simulink library "thc"  (R2021b)
settings: Solver=VariableStepAuto  StartTime=0.0  StopTime=10.0  RelTol=1e-3
undefined symbols (not defined in the file or in its folder): ATHC_APTCQA_X_C, ATHC_APTCQB_X_C, ATHC_dAy_X_C, ATHC_Qeq_X_kmh, ATHC_VbaseC_X_C, ATHC_VbaseC_Y_W, ATHC_VbaseD_X_C, ATHC_VbaseH_X_C, KTHC_ACMaxMinT_sec, KTHC_aDeice_K, KTHC_AGSDefLv_K, KTHC_AGSLv1_K, KTHC_AGSLv2_K, KTHC_AGSLv3_K, KTHC_AGSLv4_K, KTHC_AGSLv5_K, KTHC_AirIntUpdateT_sec, KTHC_APTCOneZoneMax_W, KTHC_APTCPeriod_cnt, KTHC_APTCPWMEN_flg, KTHC_APTCQMaxC_W, KTHC_APTCQminC_W, KTHC_APTCQminD_W, KTHC_APTCQminRe1_W, KTHC_APTCQminRe_W, KTHC_APTCQoffT_cnt, KTHC_APTCQonT_cnt, KTHC_APTCRiLeMaxDff_W, KTHC_APTCRiLeMinDff_W, KTHC_AutoWDTamb1_C, KTHC_AutoWDTamb2_C, KTHC_AutoWDTamb3_C, KTHC_BatCoolT_cnt, KTHC_BatInTempDef_C, KTHC_bDeice_K, KTHC_CompMaxDeice_rpm, KTHC_CompMinDeice_rpm, KTHC_CompSotxvOp_K, KTHC_CompSotxvOpLow_rpm, KTHC_CompSpdEXVUp1_rpm, KTHC_CompSpdEXVUp2_rpm, KTHC_CompSpdEXVUp3_rpm, KTHC_CompSpdEXVUp4_rpm, KTHC_CompSpdmax_rpm, KTHC_CompSpdmaxBC1_rpm, KTHC_CompSpdmaxBC_rpm, KTHC_CompSpdmid1_rpm, KTHC_CompSpdmid2_rpm, KTHC_CompSpdmid3_rpm, KTHC_CompSpdmid4_rpm, KTHC_CompSpdmid5_rpm, KTHC_CompSpdmid_rpm, KTHC_CompSpdmin_rpm, KTHC_DAPTCQ1_W, KTHC_DAPTCQ2_W, KTHC_DAPTCQ3_W, KTHC_DcChSetTemp_C, KTHC_DehumidityEN_flg, KTHC_DeiceCycTime_K, KTHC_DriveLevelWPTCBAH1_W ... (+403)
libraries: simulink x489
(part 13 of 18)

== system thc/THC/ThermalControl/THCM_Conctrl/EXV1Ctrl ==
  EXV1SHSetpoint : Inport
  PT_ Low_P1 : Inport  Port=2
  PT_ Low_T1 : Inport  Port=3
  BatteryMode : Inport  Port=4
  EXVOpen : Inport  Port=5
  ErrEXV1FroceOFF : Inport  Port=6
  HVBMTempMax : Inport  Port=7
  ChrgPlugSta : Inport  Port=8
  CompSpd : Inport  Port=9
  Chart : Stateflow chart  TreatAsAtomicUnit=on
  Compare To Constant : simulink/Logic and Bit Operations/Compare To Constant  relop===  const=1  OutDataTypeStr=boolean
  Compare To Constant1 : simulink/Logic and Bit Operations/Compare To Constant  relop===  const=1  OutDataTypeStr=boolean
  Compare To Constant2 : simulink/Logic and Bit Operations/Compare To Constant  relop===  const=6  OutDataTypeStr=boolean
  Compare To Constant3 : simulink/Logic and Bit Operations/Compare To Constant  relop===  const=6  OutDataTypeStr=boolean
  Compare To Constant4 : simulink/Logic and Bit Operations/Compare To Constant  relop===  const=2  OutDataTypeStr=boolean
  Constant : Constant  Value=0.1
  Constant1 : Constant  Value=538
  Constant{3,8..17} (11 alike) : Constant  Value=0
  Constant18 : Constant  Value=KTHC_EXVBlancePulse_K
  Constant19 : Constant  Value=ZERO_INT
  Constant2 : Constant  Value=38
  Constant20 : Constant  Value=KTHC_RefrigerantType_enum
  Constant21 : Constant  Value=KTHC_EXV1UplimLv1_K
  Constant22 : Constant  Value=KTHC_EXV1UplimLv2_K
  Constant23 : Constant  Value=KTHC_EXV1UplimLv3_K
  Constant24 : Constant  Value=KTHC_T3MinBC_C
  Constant25 : Constant  Value=KTHC_T4MinBC_C
  Constant26 : Constant  Value=KTHC_T2MaxBC_C
  Constant27 : Constant  Value=KTHC_T3MaxBC_C
  Constant28 : Constant  Value=KTHC_CompSpdEXVUp1_rpm
  Constant29 : Constant  Value=KTHC_CompSpdEXVUp2_rpm
  Constant30 : Constant  Value=KTHC_CompSpdEXVUp3_rpm
  Constant31 : Constant  Value=KTHC_CompSpdEXVUp4_rpm
  Constant4 : Constant  Value=KTHC_KpEXV1SH_K
  Constant5 : Constant  Value=KTHC_KiEXV1SHDeice_K
  Constant6 : Constant  Value=KTHC_KpEXV1SHDeice_K
  Constant7 : Constant  Value=KTHC_KiEXV1SH_K
  EXV1PIControl : Subsystem
  Equal : RelationalOperator  Operator=~=  OutDataTypeStr=boolean  RndMeth=Simplest
  Gain : Gain  Gain=1/1000
  Logical Operator : Logic  Operator=OR  AllPortsSameDT=off  OutDataTypeStr=boolean
  Logical Operator1 : Logic  AllPortsSameDT=off  OutDataTypeStr=boolean
  Logical Operator2 : Logic  Operator=OR  AllPortsSameDT=off  OutDataTypeStr=boolean
  Multiport Switch : MultiPortSwitch  Inputs=7  DiagnosticForDefault=None
  Multiport Switch1 : MultiPortSwitch  Inputs=7  DiagnosticForDefault=None
  Multiport Switch2 : MultiPortSwitch  DataPortOrder=Zero-based contiguous  zeroidx=on
  Product : Product
  R1234yf : Lookup_n-D  NumberOfTableDimensions=1  BreakpointsForDimension1=[0.03742 0.06237 0.09906 0.11778 0.15092 0.1909 0.2386 0.29495 0.36092 0.43753 0.52583 0.6269 0.74189 0.87197 1.0184 1.3023]  Table=[-50 -40 -30 -26 -20 -14 -8 -2 4 10 16 22 28 34 40 50]  InternalRulePriority=Speed  RndMeth=Simplest  InputSameDT=on
  R134a : Lookup_n-D  NumberOfTableDimensions=1  BreakpointsForDimension1=[0.02945 0.05121 0.08438 0.10167 0.13273 0.17082 0.21693 0.27217 0.33766 0.41461 0.50425 0.60789 0.72688 0.86263 1.0166 1.31790]  Table=[-50 -40 -30 -26 -20 -14 -8 -2 4 10 16 22 28 34 40 50]  InternalRulePriority=Speed  RndMeth=Simplest  InputSameDT=on
  Relational Operator : RelationalOperator  Operator=<  OutDataTypeStr=boolean  RndMeth=Simplest
  Saturation : Saturate  UpperLimit=1  LowerLimit=0
  Sum : Sum  Inputs=|-+
  Sum1 : Sum  Inputs=|+-
  Sum2 : Sum  Inputs=|+-
  Sum3 : Sum  Inputs=|++
  Switch{,1..3} (4 alike) : Switch  Criteria=u2 > Threshold
  Unit Delay : UnitDelay  SampleTime=-1  HasFrameUpgradeWarning=on
  Unit Delay1 : UnitDelay  SampleTime=-1  HasFrameUpgradeWarning=on
  EXV1 : Outport
  VTHC_EXV1P_K : Outport  Port=2
  VTHC_EXV1I_K : Outport  Port=3
  VTHC_EXV1U_K : Outport  Port=4
  VTHC_EXV1e_K : Outport  Port=5
  wires:
  Constant20/1 -> Compare To Constant4/1
  R134a/1 -> Switch2/3
  Gain/1 -> R134a/1, R1234yf/1
  Compare To Constant4/1 -> Switch2/2
  R1234yf/1 -> Switch2/1
  BatteryMode/1 -> Switch1/3
  Switch1/1 -> [BatteryMode]
  ErrEXV1FroceOFF/1 -> Switch1/2
  Constant19/1 -> Switch1/1
  Unit Delay1/1 -> Multiport Switch2/3
  EXVOpen/1 -> Multiport Switch2/1
  Constant18/1 -> Multiport Switch2/4
  Switch3/1 -> Multiport Switch2/2
  [VTHC_KiEXV1SH_K] -> EXV1PIControl/4(VTHC_KiEXV1SH_K)
  Multiport Switch1/1 -> [VTHC_KiEXV1SH_K]
  [VTHC_KpEXV1SH_K] -> EXV1PIControl/3(VTHC_KpEXV1SH_K)
  Multiport Switch/1 -> [VTHC_KpEXV1SH_K]
  Constant17/1 -> Multiport Switch1/8
  Constant16/1 -> Multiport Switch1/6
  Constant15/1 -> Multiport Switch1/5
  Constant14/1 -> Multiport Switch1/4
  Constant13/1 -> Multiport Switch1/3
  Constant12/1 -> Multiport Switch/8
  Constant11/1 -> Multiport Switch/6
  Constant10/1 -> Multiport Switch/5
  Constant9/1 -> Multiport Switch/4
  Constant8/1 -> Multiport Switch/3
  [BatteryMode] -> Multiport Switch1/1
  Constant7/1 -> Multiport Switch1/2
  Constant5/1 -> Multiport Switch1/7
  Constant6/1 -> Multiport Switch/7
  Constant4/1 -> Multiport Switch/2
  [BatteryMode] -> Multiport Switch/1
  Logical Operator2/1 -> Switch/2
  Compare To Constant3/1 -> Logical Operator2/2
  Compare To Constant1/1 -> Logical Operator2/1
  Logical Operator1/1 -> EXV1PIControl/2(Reset)
  Logical Operator/1 -> Logical Operator1/2
  Equal/1 -> Logical Operator1/1
  Compare To Constant2/1 -> Logical Operator/2
  Compare To Constant/1 -> Logical Operator/1
  Unit Delay/1 -> Equal/1
  [BatteryMode] -> Equal/2, Compare To Constant2/1, Compare To Constant/1, Unit Delay/1
  EXV1PIControl/2(VTHC_EXV1I_K) -> VTHC_EXV1I_K/1
  EXV1PIControl/1(VTHC_EXV1P_K) -> VTHC_EXV1P_K/1
  PT_ Low_T1/1 -> Sum/2  "Tlow1"
  Sum2/1 -> Saturation/1  "0.1-U"
  Constant2/1 -> Sum3/1
  Constant/1 -> Sum2/1
  Product/1 -> Sum3/2
  Saturation/1 -> Product/1  "EXV1%"
  Switch2/1 -> Sum/1  "Tsat_low1"
  EXV1SHSetpoint/1 -> Sum1/1  "SetSH"
  Multiport Switch2/1 -> EXV1/1, Unit Delay1/1  "EXV1_Pulse"
  EXV1PIControl/3(VTHC_EXV1U_K) -> Sum2/2, VTHC_EXV1U_K/1  "U"
  Sum/1 -> Sum1/2  "SH"
  PT_ Low_P1/1 -> Gain/1  "Plow1(kpa)"
  Constant3/1 -> Switch/3
  [BatteryMode] -> Compare To Constant1/1, Compare To Constant3/1
  Constant1/1 -> Product/2
  Sum1/1 -> EXV1PIControl/1(x), VTHC_EXV1e_K/1  "e"
  Sum3/1 -> Switch/1
  Relational Operator/1 -> Switch3/2
  Switch/1 -> Switch3/1, Relational Operator/1
  [VTHC_EXV1UplimPulse_K] -> Switch3/3, Relational Operator/2
  HVBMTempMax/1 -> Chart/2(HVBMTempMax)
  ChrgPlugSta/1 -> Chart/3(ChrgPlugSta)
  CompSpd/1 -> Chart/4(CompSpd)
  Constant21/1 -> Chart/5(KTHC_EXV1UplimLv1_K)
  Constant22/1 -> Chart/6(KTHC_EXV1UplimLv2_K)
  Constant23/1 -> Chart/7(KTHC_EXV1UplimLv3_K)
  Constant24/1 -> Chart/8(KTHC_T3MinBC_C)
  Constant25/1 -> Chart/9(KTHC_T4MinBC_C)
  Constant26/1 -> Chart/10(KTHC_T2MaxBC_C)
  Constant27/1 -> Chart/11(KTHC_T3MaxBC_C)
  Chart/1(VTHC_EXV1UplimPulse_K) -> [VTHC_EXV1UplimPulse_K]
  Constant28/1 -> Chart/12(KTHC_CompSpdEXVUp1_rpm)
  Constant29/1 -> Chart/13(KTHC_CompSpdEXVUp2_rpm)
  Constant30/1 -> Chart/14(KTHC_CompSpdEXVUp3_rpm)
  Constant31/1 -> Chart/15(KTHC_CompSpdEXVUp4_rpm)
  [BatteryMode] -> Chart/1(BatteryMode)

== system thc/THC/ThermalControl/THCM_Conctrl/EXV2Ctrl ==
  EXV2SHSetpoint : Inport
  PT_ Low_T2 : Inport  Port=2
  PT_ Low_P2 : Inport  Port=3
  EXV2PIDMode : Inport  Port=4
  EXVOpen : Inport  Port=5
  ErrEXV2FroceOFF : Inport  Port=6
  Compare To Constant : simulink/Logic and Bit Operations/Compare To Constant  relop=>  const=0  OutDataTypeStr=boolean
  Compare To Constant1 : simulink/Logic and Bit Operations/Compare To Constant  relop===  const=2  OutDataTypeStr=boolean
  Constant : Constant  Value=0.1
  Constant1 : Constant  Value=538
  Constant10 : Constant  Value=KTHC_EXVBlancePulse_K
  Constant11 : Constant  Value=ZERO_INT
  Constant12 : Constant  Value=KTHC_RefrigerantType_enum
  Constant2 : Constant  Value=38
  Constant3 : Constant  Value=0
  Constant4 : Constant  Value=0
  Constant5 : Constant  Value=KTHC_KpEXV2SH_K
  Constant6 : Constant  Value=KTHC_KiEXV2SH_K
  Constant7 : Constant  Value=0
  Constant8 : Constant  Value=KTHC_KpEXV2SHD_K
  Constant9 : Constant  Value=KTHC_KiEXV2SHD_K
  EXV2PIControl : Subsystem
  Gain : Gain  Gain=1/1000
  Multiport Switch : MultiPortSwitch  DataPortOrder=Zero-based contiguous  zeroidx=on
  Multiport Switch1 : MultiPortSwitch  DataPortOrder=Zero-based contiguous  zeroidx=on
  Multiport Switch2 : MultiPortSwitch  DataPortOrder=Zero-based contiguous  zeroidx=on
  Product : Product
  R1234yf : Lookup_n-D  NumberOfTableDimensions=1  BreakpointsForDimension1=[0.03742 0.06237 0.09906 0.11778 0.15092 0.1909 0.2386 0.29495 0.36092 0.43753 0.52583 0.6269 0.74189 0.87197 1.0184 1.3023]  Table=[-50 -40 -30 -26 -20 -14 -8 -2 4 10 16 22 28 34 40 50]  InternalRulePriority=Speed  RndMeth=Simplest  InputSameDT=on
  R134a : Lookup_n-D  NumberOfTableDimensions=1  BreakpointsForDimension1=[0.02945 0.05121 0.08438 0.10167 0.13273 0.17082 0.21693 0.27217 0.33766 0.41461 0.50425 0.60789 0.72688 0.86263 1.0166 1.31790]  Table=[-50 -40 -30 -26 -20 -14 -8 -2 4 10 16 22 28 34 40 50]  InternalRulePriority=Speed  RndMeth=Simplest  InputSameDT=on
  Saturation3 : Saturate  UpperLimit=1  LowerLimit=0
  Sum10 : Sum  Inputs=|++
  Sum7 : Sum  Inputs=|-+
  Sum8 : Sum  Inputs=|+-
  Sum9 : Sum  Inputs=|-+
  Switch : Switch  Criteria=u2 > Threshold
  Switch1 : Switch  Criteria=u2 > Threshold
  Switch2 : Switch  Criteria=u2 > Threshold
  Unit Delay1 : UnitDelay  SampleTime=-1  HasFrameUpgradeWarning=on
  EXV2 : Outport
  Tsat_low2 : Outport  Port=2
  VTHC_EXV2P_K : Outport  Port=3
  VTHC_EXV2I_K : Outport  Port=4
  VTHC_EXV2U_K : Outport  Port=5
  VTHC_EXV2e_K : Outport  Port=6
  wires:
  R134a/1 -> Switch2/3
  Compare To Constant1/1 -> Switch2/2
  Constant12/1 -> Compare To Constant1/1
  R1234yf/1 -> Switch2/1
  Switch1/1 -> [EXV2PIDMode]
  Constant11/1 -> Switch1/1
  ErrEXV2FroceOFF/1 -> Switch1/2
  Switch/1 -> Multiport Switch2/2
  Constant10/1 -> Multiport Switch2/4
  EXVOpen/1 -> Multiport Switch2/1
  Unit Delay1/1 -> Multiport Switch2/3
  Multiport Switch2/1 -> EXV2/1, Unit Delay1/1  "EXV2_Pulse"
  Constant3/1 -> Switch/3
  Compare To Constant/1 -> Switch/2
  [EXV2PIDMode] -> Compare To Constant/1
  [KiEXV2] -> EXV2PIControl/4(VTHC_KiEXV2_K)
  Constant9/1 -> Multiport Switch1/4
  Constant6/1 -> Multiport Switch1/3
  Multiport Switch1/1 -> [KiEXV2]
  [KpEXV2] -> EXV2PIControl/3(VTHC_KpEXV2_K)
  Constant8/1 -> Multiport Switch/4
  Constant5/1 -> Multiport Switch/3
  Multiport Switch/1 -> [KpEXV2]
  [EXV2PIDMode] -> Multiport Switch1/1
  Constant7/1 -> Multiport Switch1/2
  Constant4/1 -> Multiport Switch/2
  [EXV2PIDMode] -> Multiport Switch/1
  [EXV2PIDMode] -> EXV2PIControl/2(Reset)
  EXV2PIControl/2(VTHC_EXV2I_K) -> VTHC_EXV2I_K/1
  EXV2PIControl/1(VTHC_EXV2P_K) -> VTHC_EXV2P_K/1
  Product/1 -> Sum10/2
  Sum8/1 -> EXV2PIControl/1(x), VTHC_EXV2e_K/1  "e"
  Switch2/1 -> Sum7/1, Tsat_low2/1  "Tsat_low2"
  EXV2SHSetpoint/1 -> Sum8/1
  PT_ Low_P2/1 -> Gain/1
  EXV2PIDMode/1 -> Switch1/3
  Sum10/1 -> Switch/1  "EXV2_Pulse"
  PT_ Low_T2/1 -> Sum7/2  "Tlow2"
  Sum7/1 -> Sum8/2  "SH"
  Constant2/1 -> Sum10/1
  Saturation3/1 -> Product/1  "EXV2%"
  Gain/1 -> R134a/1, R1234yf/1
  Sum9/1 -> Saturation3/1  "0.1-U"
  Constant1/1 -> Product/2
  Constant/1 -> Sum9/2
  EXV2PIControl/3(VTHC_EXV2U_K) -> Sum9/1, VTHC_EXV2U_K/1  "U"

== system thc/THC/ThermalControl/THCM_Conctrl/RadiatorFan ==
  FAN : Inport
  AGS_Err : Inport  Port=2
  AGS : Inport  Port=3
  Compare To Constant : simulink/Logic and Bit Operations/Compare To Constant  relop=>  const=1  OutDataTypeStr=boolean
  Constant : Constant  Value=KTHC_FANLv1_pct
  Constant1 : Constant  Value=KTHC_FANLv2_pct
  Constant2 : Constant  Value=KTHC_FANLv3_pct
  Constant3 : Constant  Value=KTHC_FANLv4_pct
  Constant4 : Constant  Value=KTHC_FANLv5_pct
  Constant5 : Constant  Value=0
  Constant6 : Constant  Value=KTHC_FANDefLv_pct
  Constant7 : Constant  Value=KTHC_ErrHandleEN_flg
  Logical Operator : Logic  Inputs=3  AllPortsSameDT=off  OutDataTypeStr=boolean
  Multiport Switch : MultiPortSwitch  Inputs=6  DiagnosticForDefault=None
  Switch : Switch  Criteria=u2 > Threshold
  CoolgFanActDuty : Outport
  wires:
  Constant7/1 -> Logical Operator/3
  Multiport Switch/1 -> Switch/3
  Switch/1 -> CoolgFanActDuty/1
  Compare To Constant/1 -> Logical Operator/2
  AGS_Err/1 -> Logical Operator/1
  AGS/1 -> Compare To Constant/1
  Constant6/1 -> Switch/1
  Logical Operator/1 -> Switch/2
  Constant3/1 -> Multiport Switch/5
  Constant2/1 -> Multiport Switch/4
  Constant1/1 -> Multiport Switch/3
  Constant4/1 -> Multiport Switch/6
  Constant5/1 -> Multiport Switch/7
  Constant/1 -> Multiport Switch/2
  FAN/1 -> Multiport Switch/1

== system thc/THC/ThermalControl/THCM_Conctrl/SensorErrorHandle1 ==
  DataIn : Inport
  SensorError : Inport  Port=2
  PresetValue : Inport  Port=3
  Constant : Constant  Value=KTHC_ErrHandleEN_flg
  Logical Operator : Logic  AllPortsSameDT=off  OutDataTypeStr=boolean
  Switch : Switch  Criteria=u2 > Threshold
  DataOut : Outport
  wires:
  Constant/1 -> Logical Operator/2
  SensorError/1 -> Logical Operator/1
  Logical Operator/1 -> Switch/2
  Switch/1 -> DataOut/1
  DataIn/1 -> Switch/3
  PresetValue/1 -> Switch/1

== system thc/THC/ThermalControl/THCM_Conctrl/SensorErrorHandle10 ==
  DataIn : Inport
  SensorError : Inport  Port=2
  PresetValue : Inport  Port=3
  Constant : Constant  Value=KTHC_ErrHandleEN_flg
  Logical Operator : Logic  AllPortsSameDT=off  OutDataTypeStr=boolean
  Switch : Switch  Criteria=u2 > Threshold
  DataOut : Outport
  wires:
  PresetValue/1 -> Switch/1
  DataIn/1 -> Switch/3
  Switch/1 -> DataOut/1
  Logical Operator/1 -> Switch/2
  SensorError/1 -> Logical Operator/1
  Constant/1 -> Logical Operator/2

== system thc/THC/ThermalControl/THCM_Conctrl/SensorErrorHandle11 ==
  DataIn : Inport
  SensorError : Inport  Port=2
  PresetValue : Inport  Port=3
  Constant : Constant  Value=KTHC_ErrHandleEN_flg
  Logical Operator : Logic  AllPortsSameDT=off  OutDataTypeStr=boolean
  Switch : Switch  Criteria=u2 > Threshold
  DataOut : Outport
  wires:
  PresetValue/1 -> Switch/1
  DataIn/1 -> Switch/3
  Switch/1 -> DataOut/1
  Logical Operator/1 -> Switch/2
  SensorError/1 -> Logical Operator/1
  Constant/1 -> Logical Operator/2

== system thc/THC/ThermalControl/THCM_Conctrl/SensorErrorHandle12 ==
  DataIn : Inport
  SensorError : Inport  Port=2
  PresetValue : Inport  Port=3
  Constant : Constant  Value=KTHC_ErrHandleEN_flg
  Logical Operator : Logic  AllPortsSameDT=off  OutDataTypeStr=boolean
  Switch : Switch  Criteria=u2 > Threshold
  DataOut : Outport
  wires:
  PresetValue/1 -> Switch/1
  DataIn/1 -> Switch/3
  Switch/1 -> DataOut/1
  Logical Operator/1 -> Switch/2
  SensorError/1 -> Logical Operator/1
  Constant/1 -> Logical Operator/2

== system thc/THC/ThermalControl/THCM_Conctrl/SensorErrorHandle2 ==
  DataIn : Inport
  SensorError : Inport  Port=2
  PresetValue : Inport  Port=3
  Constant : Constant  Value=KTHC_ErrHandleEN_flg
  Logical Operator : Logic  AllPortsSameDT=off  OutDataTypeStr=boolean
  Switch : Switch  Criteria=u2 > Threshold
  DataOut : Outport
  wires:
  PresetValue/1 -> Switch/1
  DataIn/1 -> Switch/3
  Switch/1 -> DataOut/1
  Logical Operator/1 -> Switch/2
  SensorError/1 -> Logical Operator/1
  Constant/1 -> Logical Operator/2

== system thc/THC/ThermalControl/THCM_Conctrl/SensorErrorHandle3 ==
  DataIn : Inport
  SensorError : Inport  Port=2
  PresetValue : Inport  Port=3
  Constant : Constant  Value=KTHC_ErrHandleEN_flg
  Logical Operator : Logic  AllPortsSameDT=off  OutDataTypeStr=boolean
  Switch : Switch  Criteria=u2 > Threshold
  DataOut : Outport
  wires:
  Constant/1 -> Logical Operator/2
  SensorError/1 -> Logical Operator/1
  Logical Operator/1 -> Switch/2
  Switch/1 -> DataOut/1
  DataIn/1 -> Switch/3
  PresetValue/1 -> Switch/1

== system thc/THC/ThermalControl/THCM_Conctrl/SensorErrorHandle4 ==
  DataIn : Inport
  SensorError : Inport  Port=2
  PresetValue : Inport  Port=3
  Constant : Constant  Value=KTHC_TevaErrHandleEN_flg
  Logical Operator : Logic  AllPortsSameDT=off  OutDataTypeStr=boolean
  Switch : Switch  Criteria=u2 > Threshold
  DataOut : Outport
  wires:
  Constant/1 -> Logical Operator/2
  SensorError/1 -> Logical Operator/1
  Logical Operator/1 -> Switch/2
  Switch/1 -> DataOut/1
  DataIn/1 -> Switch/3
  PresetValue/1 -> Switch/1

== system thc/THC/ThermalControl/THCM_Conctrl/SensorErrorHandle5 ==
  DataIn : Inport
  SensorError : Inport  Port=2
  PresetValue : Inport  Port=3
  Constant : Constant  Value=KTHC_TevaErrHandleEN_flg
  Logical Operator : Logic  AllPortsSameDT=off  OutDataTypeStr=boolean
  Switch : Switch  Criteria=u2 > Threshold
  DataOut : Outport
  wires:
  PresetValue/1 -> Switch/1
  DataIn/1 -> Switch/3
  Switch/1 -> DataOut/1
  Logical Operator/1 -> Switch/2
  SensorError/1 -> Logical Operator/1
  Constant/1 -> Logical Operator/2

== system thc/THC/ThermalControl/THCM_Conctrl/SensorErrorHandle6 ==
  DataIn : Inport
  SensorError : Inport  Port=2
  PresetValue : Inport  Port=3
  Constant : Constant  Value=KTHC_TevaErrHandleEN_flg
  Logical Operator : Logic  AllPortsSameDT=off  OutDataTypeStr=boolean
  Switch : Switch  Criteria=u2 > Threshold
  DataOut : Outport
  wires:
  Constant/1 -> Logical Operator/2
  SensorError/1 -> Logical Operator/1
  Logical Operator/1 -> Switch/2
  Switch/1 -> DataOut/1
  DataIn/1 -> Switch/3
  PresetValue/1 -> Switch/1

== system thc/THC/ThermalControl/THCM_Conctrl/SensorErrorHandle7 ==
  DataIn : Inport
  SensorError : Inport  Port=2
  PresetValue : Inport  Port=3
  Constant : Constant  Value=KTHC_TevaErrHandleEN_flg
  Logical Operator : Logic  AllPortsSameDT=off  OutDataTypeStr=boolean
  Switch : Switch  Criteria=u2 > Threshold
  DataOut : Outport
  wires:
  PresetValue/1 -> Switch/1
  DataIn/1 -> Switch/3
  Switch/1 -> DataOut/1
  Logical Operator/1 -> Switch/2
  SensorError/1 -> Logical Operator/1
  Constant/1 -> Logical Operator/2

== system thc/THC/ThermalControl/THCM_Conctrl/SensorErrorHandle8 ==
  DataIn : Inport
  SensorError : Inport  Port=2
  PresetValue : Inport  Port=3
  Constant : Constant  Value=KTHC_TevaErrHandleEN_flg
  Logical Operator : Logic  AllPortsSameDT=off  OutDataTypeStr=boolean
  Switch : Switch  Criteria=u2 > Threshold
  DataOut : Outport
  wires:
  Constant/1 -> Logical Operator/2
  SensorError/1 -> Logical Operator/1
  Logical Operator/1 -> Switch/2
  Switch/1 -> DataOut/1
  DataIn/1 -> Switch/3
  PresetValue/1 -> Switch/1

== system thc/THC/ThermalControl/THCM_Conctrl/SensorErrorHandle9 ==
  DataIn : Inport
  SensorError : Inport  Port=2
  PresetValue : Inport  Port=3
  Constant : Constant  Value=KTHC_TevaErrHandleEN_flg
  Logical Operator : Logic  AllPortsSameDT=off  OutDataTypeStr=boolean
  Switch : Switch  Criteria=u2 > Threshold
  DataOut : Outport
  wires:
  PresetValue/1 -> Switch/1
  DataIn/1 -> Switch/3
  Switch/1 -> DataOut/1
  Logical Operator/1 -> Switch/2
  SensorError/1 -> Logical Operator/1
  Constant/1 -> Logical Operator/2

== system thc/THC/ThermalControl/THCM_Conctrl/Subsystem ==
  CompSpd : Inport
  CabinMode : Inport  Port=2
  CompFB : Inport  Port=3
  Chart : Stateflow chart  TreatAsAtomicUnit=on
      settings: PortSchema="{\"entries\":[{\"content\":{\"sides\":[{\"content\":{\"connectorIds\":[\"In7\",\"In1\",\"In2\",\"In3\",\"In4\",\"In5\",\"In6\",\"In8\",\"In9\",\"In10\",\"In11\"]},\"type\":\"ConnectorPlacement.EquallySpacedRectSide\",\"uuid\":\"1db6d48d-2993-4fd1-a317-039acf53791d\"},{\"content\":{\"connectorIds\":[\"Out1\",\"Out2\",\"Out3\"],\"side\":\"RIGHT\"},\"type\":\"ConnectorPlacement.EquallySpacedRectSide\",\"uuid\":\"3b07bc2c-8788-4d9a-bac7-12ac97bb3dfe\"},{\"content\":{\"connectorIds\":[],\"side\":\"TOP\"},\"type\":\"ConnectorPlacement.EquallySpacedRectSide\",\"uuid\":\"678ef0de-745c-42f5-bb8c-af17f8a0632e\"}]},\"type\":\"ConnectorPlacement.EquallySpacedConnector\",\"uuid\":\"729d42ab-7bc1-4f80-88b9-90079b8c4930\"}],\"packageUris\":[\"http://schema.mathworks.com/mf0/Connector/R2020b\"],\"version\":\"1.0\"}"
  Compare To Constant : simulink/Logic and Bit Operations/Compare To Constant  relop=>=  const=2  OutDataTypeStr=boolean
  Compare To Constant1 : simulink/Logic and Bit Operations/Compare To Constant  relop=>  const=3  OutDataTypeStr=boolean
  Compare To Constant10 : simulink/Logic and Bit Operations/Compare To Constant  relop=<  const=10  OutDataTypeStr=boolean
  Compare To Constant11 : simulink/Logic and Bit Operations/Compare To Constant  relop===  const=9  OutDataTypeStr=boolean
  Compare To Constant12 : simulink/Logic and Bit Operations/Compare To Constant  relop===  const=1  OutDataTypeStr=boolean
  Compare To Constant13 : simulink/Logic and Bit Operations/Compare To Constant  relop===  const=5  OutDataTypeStr=boolean
  Compare To Constant2 : simulink/Logic and Bit Operations/Compare To Constant  relop=>=  const=1  OutDataTypeStr=boolean
  Compare To Constant3 : simulink/Logic and Bit Operations/Compare To Constant  relop=<=  const=3  OutDataTypeStr=boolean
  Compare To Constant4 : simulink/Logic and Bit Operations/Compare To Constant  relop===  const=8  OutDataTypeStr=boolean
  Compare To Constant5 : simulink/Logic and Bit Operations/Compare To Constant  relop===  const=6  OutDataTypeStr=boolean
  Compare To Constant6 : simulink/Logic and Bit Operations/Compare To Constant  relop===  const=7  OutDataTypeStr=boolean
  Compare To Constant7 : simulink/Logic and Bit Operations/Compare To Constant  relop===  const=4  OutDataTypeStr=boolean
  Compare To Constant8 : simulink/Logic and Bit Operations/Compare To Constant  relop=~=  const=7  OutDataTypeStr=boolean
  Compare To Constant9 : simulink/Logic and Bit Operations/Compare To Constant  relop=>=  const=10  OutDataTypeStr=boolean
  Constant3 : Constant  Value=0
  Constant4 : Constant  Value=KTHC_PBlaceTime1_K
  Constant5 : Constant  Value=KTHC_PBlaceTime2_K
  Constant6 : Constant  Value=KTHC_PBlaceTime3_K
  Constant7 : Constant  Value=KTHC_PBlaceTime4_K
  Logical Operator : Logic  AllPortsSameDT=off  OutDataTypeStr=boolean
  Logical Operator1 : Logic  Operator=OR  Inputs=4  AllPortsSameDT=off  OutDataTypeStr=boolean
  Logical Operator2 : Logic  Operator=OR  Inputs=4  AllPortsSameDT=off  OutDataTypeStr=boolean
  Logical Operator3 : Logic  Operator=OR  AllPortsSameDT=off  OutDataTypeStr=boolean
  Logical Operator4 : Logic  Inputs=3  AllPortsSameDT=off  OutDataTypeStr=boolean
  Logical Operator7 : Logic  Operator=NOT  AllPortsSameDT=off  OutDataTypeStr=boolean
  Logical Operator8 : Logic  AllPortsSameDT=off  OutDataTypeStr=boolean
  NOT : Logic  Operator=NOT  IconShape=distinctive  AllPortsSameDT=off  OutDataTypeStr=boolean
  NOT1 : Logic  Operator=NOT  IconShape=distinctive  AllPortsSameDT=off  OutDataTypeStr=boolean
  NOT2 : Logic  Operator=NOT  IconShape=distinctive  AllPortsSameDT=off  OutDataTypeStr=boolean
  Switch{,2,4,6} (4 alike) : Switch  Criteria=u2 > Threshold
  Unit Delay{,1..5} (6 alike) : UnitDelay  SampleTime=-1  HasFrameUpgradeWarning=on
  FD_Comp_Cmd : Outport
  FD_SOV1_Cmd : Outport  Port=2
  FD_SOV2_Cmd : Outport  Port=3
  FD_SOV3_Cmd : Outport  Port=4
  EXVOpen : Outport  Port=5
  wires:
  Compare To Constant4/1 -> Logical Operator2/1
  Compare To Constant11/1 -> Logical Operator2/2
  Constant7/1 -> Chart/11(KTHC_PBlaceTime4_K)
  Chart/3(EXVOpen) -> EXVOpen/1
  Constant6/1 -> Chart/10(KTHC_PBlaceTime3_K)
  Constant5/1 -> Chart/9(KTHC_PBlaceTime2_K)
  Constant4/1 -> Chart/8(KTHC_PBlaceTime1_K)
  Compare To Constant13/1 -> Logical Operator2/4
  Compare To Constant10/1 -> Logical Operator4/3
  Compare To Constant9/1 -> Logical Operator1/4
  Compare To Constant8/1 -> Logical Operator4/2
  Logical Operator4/1 -> Logical Operator3/2
  Compare To Constant7/1 -> Logical Operator2/3
  CabinMode/1 -> Compare To Constant3/1, Compare To Constant2/1, Compare To Constant/1, Compare To Constant6/1, Compare To Constant12/1, Compare To Constant1/1, Compare To Constant8/1, Compare To Constant10/1, Compare To Constant4/1, Compare To Constant13/1, Compare To Constant7/1, Compare To Constant11/1, Compare To Constant9/1, Compare To Constant5/1
  Compare To Constant6/1 -> Logical Operator1/3
  Compare To Constant5/1 -> Logical Operator1/2
  Logical Operator/1 -> Logical Operator1/1
  Compare To Constant/1 -> Logical Operator8/1
  CompFB/1 -> Chart/7(Comp)
  Compare To Constant1/1 -> Logical Operator4/1
  Compare To Constant2/1 -> Logical Operator/1
  Compare To Constant3/1 -> Logical Operator/2
  Compare To Constant12/1 -> Logical Operator3/1
  Chart/1(FCompOFF) -> Logical Operator7/1
  Logical Operator8/1 -> Switch6/2
  Constant3/1 -> Switch6/3
  Switch6/1 -> FD_Comp_Cmd/1  "FD_Comp_Cmd"
  CompSpd/1 -> Switch6/1
  Logical Operator7/1 -> Logical Operator8/2
  NOT2/1 -> FD_SOV3_Cmd/1  "FD_SOV3_Cmd"
  NOT1/1 -> FD_SOV2_Cmd/1  "FD_SOV2_Cmd"
  NOT/1 -> FD_SOV1_Cmd/1  "FD_SOV1_Cmd"
  [Keep] -> Switch4/2
  [SOV3C] -> Switch4/3
  Switch4/1 -> NOT2/1, Unit Delay5/1
  Unit Delay5/1 -> Switch4/1
  Unit Delay4/1 -> Switch2/1
  Switch2/1 -> NOT1/1, Unit Delay4/1
  [SOV2C] -> Switch2/3
  [Keep] -> Switch2/2
  [Keep] -> Switch/2
  [SOV1C] -> Switch/3
  Chart/2(Keep) -> [Keep]
  Switch/1 -> NOT/1, Unit Delay3/1
  Unit Delay3/1 -> Switch/1
  Unit Delay2/1 -> Chart/6(SOV3CBuf)
  Logical Operator2/1 -> Unit Delay2/1, Chart/5(SOV3C), [SOV3C]
  Logical Operator3/1 -> Chart/3(SOV2C), [SOV2C], Unit Delay1/1
  Unit Delay1/1 -> Chart/4(SOV2CBuf)
  Unit Delay/1 -> Chart/2(SOV1CBuf)
  Logical Operator1/1 -> Chart/1(SOV1C), [SOV1C], Unit Delay/1

== system thc/THC/ThermalControl/THCM_Conctrl/Subsystem1 ==
  T_Face_L : Inport
  T_Face_R : Inport  Port=2
  T_Foot_L : Inport  Port=3
  T_Foot_R : Inport  Port=4
  T_Face_Rr : Inport  Port=5
  T_Foot_Rr : Inport  Port=6
  T_Face_L_Err : Inport  Port=7
  T_Face_R_Err : Inport  Port=8
  T_Foot_L_Err : Inport  Port=9
  T_Foot_R_Err : Inport  Port=10
  T_Face_Rr_Err : Inport  Port=11
  T_Foot_Rr_Err : Inport  Port=12
  CabinMode : Inport  Port=13
  Tincar : Inport  Port=14
  Tincar_Err : Inport  Port=15
  ACSubMode : Inport  Port=16
  Add : Sum  Inputs=++++++
  Add1 : Sum  Inputs=++++++
  Add2 : Sum
  Compare To Constant : simulink/Logic and Bit Operations/Compare To Constant  relop=<  const=4  OutDataTypeStr=boolean
  Compare To Constant1 : simulink/Logic and Bit Operations/Compare To Constant  relop=<  const=8  OutDataTypeStr=boolean
  Compare To Constant2 : simulink/Logic and Bit Operations/Compare To Constant  relop=~=  const=0  OutDataTypeStr=boolean
  Compare To Constant3 : simulink/Logic and Bit Operations/Compare To Constant  relop===  const=6  OutDataTypeStr=boolean
  Compare To Constant4 : simulink/Logic and Bit Operations/Compare To Constant  relop===  const=2  OutDataTypeStr=boolean
  Constant1 : Constant  Value=KTHC_TdiffC_C
  Constant{134..139} (6 alike) : Constant  Value=0
  Constant2 : Constant  Value=KTHC_TdiffD_C
  Constant3 : Constant  Value=KTHC_TdiffH_C
  Constant4 : Constant  Value=KTHC_TductDef_C
  Data Type Conversion{,1..7} (8 alike) : DataTypeConversion
  Divide : Product  Inputs=*/
  Logical Operator : Logic  Operator=OR  AllPortsSameDT=off  OutDataTypeStr=boolean
  Logical Operator1 : Logic  AllPortsSameDT=off  OutDataTypeStr=boolean
  NOT{,1..5} (6 alike) : Logic  Operator=NOT  IconShape=distinctive  AllPortsSameDT=off  OutDataTypeStr=boolean
  SensorErrorHandle1 : Subsystem
  SensorErrorHandle2 : Subsystem
  SensorErrorHandle3 : Subsystem
  SensorErrorHandle4 : Subsystem
  SensorErrorHandle5 : Subsystem
  SensorErrorHandle9 : Subsystem
  Switch{,1..3} (4 alike) : Switch  Criteria=u2 > Threshold
  Unit Delay : UnitDelay  SampleTime=-1  HasFrameUpgradeWarning=on
  Unit Delay1 : UnitDelay  SampleTime=-1  HasFrameUpgradeWarning=on
  TincarFix : Outport
  wires:
  Unit Delay1/1 -> Compare To Constant4/1
  Compare To Constant3/1 -> Logical Operator1/2
  Logical Operator1/1 -> Logical Operator/1
  Compare To Constant4/1 -> Logical Operator1/1
  ACSubMode/1 -> Unit Delay1/1
  Logical Operator/1 -> Switch/2
  Compare To Constant/1 -> Logical Operator/2
  Data Type Conversion7/1 -> Switch2/1
  Data Type Conversion6/1 -> Switch3/1
  Switch3/1 -> TincarFix/1
  Tincar/1 -> Switch3/3
  Add2/1 -> Data Type Conversion6/1
  Tincar_Err/1 -> Switch3/2
  Switch/1 -> Add2/2
  Switch2/1 -> Add2/1
  Constant4/1 -> Switch2/3
  Divide/1 -> Data Type Conversion7/1
  Compare To Constant2/1 -> Switch2/2
  Constant3/1 -> Switch1/3
  Constant2/1 -> Switch1/1
  Constant1/1 -> Switch/1
  Compare To Constant1/1 -> Switch1/2
  Switch1/1 -> Switch/3
  Unit Delay/1 -> Compare To Constant/1, Compare To Constant1/1, Compare To Constant3/1
  CabinMode/1 -> Unit Delay/1
  Add1/1 -> Divide/2, Compare To Constant2/1
  Add/1 -> Divide/1
  NOT5/1 -> Data Type Conversion5/1
  [T_Foot_Rr_Err] -> NOT5/1
  Data Type Conversion5/1 -> Add1/6
  Data Type Conversion4/1 -> Add1/5
  [T_Face_Rr_Err] -> NOT4/1
  NOT4/1 -> Data Type Conversion4/1
  NOT3/1 -> Data Type Conversion3/1
  [T_Foot_R_Err] -> NOT3/1
  Data Type Conversion3/1 -> Add1/4
  Data Type Conversion2/1 -> Add1/3
  [T_Foot_L_Err] -> NOT2/1
  NOT2/1 -> Data Type Conversion2/1
  Data Type Conversion1/1 -> Add1/2
  NOT1/1 -> Data Type Conversion1/1
  [T_Face_R_Err] -> NOT1/1
  [T_Face_L_Err] -> NOT/1
  NOT/1 -> Data Type Conversion/1
  Data Type Conversion/1 -> Add1/1
  SensorErrorHandle4/1(DataOut) -> Add/2
  SensorErrorHandle3/1(DataOut) -> Add/3
  SensorErrorHandle1/1(DataOut) -> Add/5
  SensorErrorHandle2/1(DataOut) -> Add/4
  SensorErrorHandle9/1(DataOut) -> Add/6
  SensorErrorHandle5/1(DataOut) -> Add/1
  Constant139/1 -> SensorErrorHandle9/3(PresetValue)
  [T_Foot_Rr_Err] -> SensorErrorHandle9/2(SensorError)
  Constant138/1 -> SensorErrorHandle1/3(PresetValue)
  [T_Face_Rr_Err] -> SensorErrorHandle1/2(SensorError)
  T_Face_L/1 -> SensorErrorHandle5/1(DataIn)
  Constant134/1 -> SensorErrorHandle5/3(PresetValue)
  [T_Face_L_Err] -> SensorErrorHandle5/2(SensorError)
  Constant137/1 -> SensorErrorHandle2/3(PresetValue)
  [T_Foot_R_Err] -> SensorErrorHandle2/2(SensorError)
  Constant136/1 -> SensorErrorHandle3/3(PresetValue)
  [T_Foot_L_Err] -> SensorErrorHandle3/2(SensorError)
  Constant135/1 -> SensorErrorHandle4/3(PresetValue)
  [T_Face_R_Err] -> SensorErrorHandle4/2(SensorError)
  T_Face_L_Err/1 -> [T_Face_L_Err]
  T_Face_Rr_Err/1 -> [T_Face_Rr_Err]
  T_Foot_Rr_Err/1 -> [T_Foot_Rr_Err]
  T_Foot_Rr/1 -> SensorErrorHandle9/1(DataIn)
  T_Face_Rr/1 -> SensorErrorHandle1/1(DataIn)
  T_Face_R_Err/1 -> [T_Face_R_Err]
  T_Foot_L/1 -> SensorErrorHandle3/1(DataIn)
  T_Foot_R/1 -> SensorErrorHandle2/1(DataIn)
  T_Foot_R_Err/1 -> [T_Foot_R_Err]
  T_Face_R/1 -> SensorErrorHandle4/1(DataIn)
  T_Foot_L_Err/1 -> [T_Foot_L_Err]

== system thc/THC/ThermalControl/THCM_Conctrl/Subsystem2 ==
  Motor_In_Temp : Inport
  Motor_In_Temp_Err : Inport  Port=2
  TBMax : Inport  Port=3
  Compare To Constant : simulink/Logic and Bit Operations/Compare To Constant  relop=>  const=20  OutDataTypeStr=boolean
  Constant1 : Constant  Value=KTHC_MotorInTempDefL_C
  Constant140 : Constant  Value=KTHC_MotorInTempDefH_C
  SensorErrorHandle9 : Subsystem
  Switch : Switch  Criteria=u2 > Threshold
  Motor_In_TempFix : Outport
  wires:
  SensorErrorHandle9/1(DataOut) -> Motor_In_TempFix/1
  Switch/1 -> SensorErrorHandle9/3(PresetValue)
  Motor_In_Temp_Err/1 -> SensorErrorHandle9/2(SensorError)
  Motor_In_Temp/1 -> SensorErrorHandle9/1(DataIn)
  Constant1/1 -> Switch/3
  Constant140/1 -> Switch/1
  Compare To Constant/1 -> Switch/2
  TBMax/1 -> Compare To Constant/1

== system thc/THC/ThermalControl/THCM_Conctrl/Subsystem3 ==
  note: 50
  FWVin : Inport
  TWVin : Inport  Port=2
  EWP1in : Inport  Port=3
  EWP2in : Inport  Port=4
  EWP3in : Inport  Port=5
  BalanceSW : Inport  Port=6
  "VINP_EWP1BlockError_enum " : Inport  Port=7
  VINP_EWP1OverCurrError_enum : Inport  Port=8
  VINP_EWP2BlockError_enum : Inport  Port=9
  VINP_EWP2OverCurrError_enum : Inport  Port=10
  VINP_EWP3BlockError_enum : Inport  Port=11
  VINP_EWP3OverCurrError_enum : Inport  Port=12
  Chart : Stateflow chart  TreatAsAtomicUnit=on
  Constant : Constant  Value=240
  Constant1 : Constant  Value=KTHC_ValueSWT_cnt
  Constant2 : Constant
  Constant3 : Constant  Value=0
  Constant4 : Constant  Value=0
  Constant5 : Constant  Value=0
  Constant9 : Constant  Value=KTHC_EWPStopT_cnt
  Data Type Conversion{,1..2,4..7} (7 alike) : DataTypeConversion  OutDataTypeStr=uint8
  Data Type Conversion3 : DataTypeConversion  OutDataTypeStr=boolean
  Detect Change : simulink/Logic and Bit Operations/Detect Change  vinit=0  OutDataTypeStr=boolean
  Detect Change1 : simulink/Logic and Bit Operations/Detect Change  vinit=0  OutDataTypeStr=boolean
  Logical Operator{,2,5..10} (8 alike) : Logic  AllPortsSameDT=off  OutDataTypeStr=boolean
  Logical Operator1 : Logic  Operator=OR  AllPortsSameDT=off  OutDataTypeStr=boolean
  Logical Operator11 : Logic  Operator=OR  Inputs=3  AllPortsSameDT=off  OutDataTypeStr=boolean
  Logical Operator3 : Logic  Operator=NOT  AllPortsSameDT=off  OutDataTypeStr=boolean
  Logical Operator4 : Logic  Operator=OR  AllPortsSameDT=off  OutDataTypeStr=boolean
  Max : MinMax  Function=max  Inputs=3
  Subsystem1 : Subsystem
  Subsystem2 : Subsystem
  Subsystem3 : Subsystem
  Switch{,1..12} (13 alike) : Switch  Criteria=u2 > Threshold
  Unit Delay{,1..7} (8 alike) : UnitDelay  SampleTime=-1  HasFrameUpgradeWarning=on
  FWV : Outport
  TWV : Outport  Port=2
  EWP1 : Outport  Port=3
  EWP2 : Outport  Port=4
  EWP3 : Outport  Port=5
  VTHC_EWPBUflag1_flg : Outport  Port=6
  VTHC_EWPBUflag2_flg : Outport  Port=7
  VTHC_EWPBUflag3_flg : Outport  Port=8
  VTHC_THSysErrlampReq_flg : Outport  Port=9
  wires:
  [EWP2in] -> Max/2
  [FWVin] -> Switch1/3
  Switch1/1 -> Unit Delay4/1, [FWV]
  Unit Delay4/1 -> Switch1/1
  [FWVin] -> Detect Change/1, Logical Operator/1
  [EWPMax] -> Switch7/1
  [EWP3in] -> Switch7/3
  [EWPMax] -> Switch3/1
  Unit Delay3/1 -> Switch/1
  [EWP1in] -> Max/1
  Constant9/1 -> Data Type Conversion/1
  TWVin/1 -> [TWVin]
  Logical Operator1/1 -> [AllStopReq]
  Chart/2(FWVKeep) -> [FWVKeep]
  Logical Operator7/1 -> Switch7/2, Switch3/2, Switch2/2
  Unit Delay1/1 -> Chart/4(EWP2)
  [EWP1in] -> Switch2/3
  Switch8/1 -> [EWPMax]
  FWVin/1 -> Switch9/3
  [EWP3in] -> Max/3
  [EWPMax] -> Switch2/1
  Logical Operator2/1 -> [PartStopReq]
  Detect Change1/1 -> Logical Operator2/1, Logical Operator/2
  [EWP2] -> Unit Delay1/1
  Switch2/1 -> Switch4/3
  Logical Operator/1 -> Logical Operator1/2
  [TWVin] -> Switch/3
  [EWP2in] -> Switch3/3
  [TWVin] -> Data Type Conversion4/1
  Unit Delay2/1 -> Chart/3(EWP1)
  Unit Delay/1 -> Chart/5(EWP3)
  [FWVin] -> Logical Operator3/1
  Logical Operator3/1 -> Logical Operator2/2
  Data Type Conversion/1 -> Chart/6(EWPStopT)
  Detect Change/1 -> Logical Operator1/1
  [EWP3] -> Unit Delay/1
  Chart/1(TWVKeep) -> [TWVKeep]
  Switch/1 -> TWV/1, Unit Delay3/1
  [EWP1] -> Unit Delay2/1
  [FWV] -> FWV/1
  [FWVin] -> Logical Operator4/1
  [FWV] -> Logical Operator4/2
  [PartStopReq] -> Chart/1(PartStopReq)
  [AllStopReq] -> Chart/2(AllStopReq)
  EWP1in/1 -> [EWP1in]
  EWP2in/1 -> [EWP2in]
  EWP3in/1 -> [EWP3in]
  Constant1/1 -> Data Type Conversion1/1
  Data Type Conversion1/1 -> Chart/7(ValueSWT)
  Chart/3(EWPKeep) -> [EWPKeep]
  Unit Delay5/1 -> Switch4/1
  Switch4/1 -> Unit Delay5/1, [EWP1]
  Switch5/1 -> [EWP2], Unit Delay6/1
  Unit Delay6/1 -> Switch5/1
  Switch3/1 -> Switch5/3
  Switch7/1 -> Switch6/3
  Unit Delay7/1 -> Switch6/1
  Switch6/1 -> [EWP3], Unit Delay7/1
  BalanceSW/1 -> [BalanceSW]
  Logical Operator5/1 -> Switch/2
  [BalanceSW] -> Logical Operator5/1
  [TWVKeep] -> Logical Operator5/2
  Logical Operator6/1 -> Switch1/2
  [FWVKeep] -> Logical Operator6/2
  [BalanceSW] -> Logical Operator6/1
  Logical Operator4/1 -> Logical Operator7/2
  [BalanceSW] -> Logical Operator7/1
  Logical Operator8/1 -> Switch4/2
  [EWPKeep] -> Logical Operator8/2
  [BalanceSW] -> Logical Operator8/1
  Logical Operator9/1 -> Switch5/2
  [EWPKeep] -> Logical Operator9/2
  [BalanceSW] -> Logical Operator9/1
  Logical Operator10/1 -> Switch6/2
  [EWPKeep] -> Logical Operator10/2
  [BalanceSW] -> Logical Operator10/1
  Subsystem3/1(EWPerror) -> [EWP1error]
  "VINP_EWP1BlockError_enum "/1 -> Subsystem3/1("VINP_EWPBlockError_enum ")
  VINP_EWP1OverCurrError_enum/1 -> Subsystem3/2(VINP_EWPOverCurrError_enum)
  VINP_EWP2BlockError_enum/1 -> Subsystem1/1("VINP_EWPBlockError_enum ")
  VINP_EWP2OverCurrError_enum/1 -> Subsystem1/2(VINP_EWPOverCurrError_enum)
  VINP_EWP3BlockError_enum/1 -> Subsystem2/1("VINP_EWPBlockError_enum ")
  VINP_EWP3OverCurrError_enum/1 -> Subsystem2/2(VINP_EWPOverCurrError_enum)
  Subsystem1/1(EWPerror) -> [EWP2error]
  Subsystem2/1(EWPerror) -> [EWP3error]
  [EWP1error] -> Logical Operator11/1
  [EWP2error] -> Logical Operator11/2
  [EWP3error] -> Logical Operator11/3
  Logical Operator11/1 -> [FWVForceON]
  Max/1 -> Switch8/3
  [FWVForceON] -> Switch8/2
  Data Type Conversion2/1 -> Switch8/1
  Constant/1 -> Data Type Conversion2/1
  Switch9/1 -> [FWVin]
  [FWVForceON] -> Switch9/2
  Data Type Conversion3/1 -> Switch9/1
  Constant2/1 -> Data Type Conversion3/1
  Data Type Conversion4/1 -> Detect Change1/1
  Subsystem3/2(EWPpause) -> [EWP1pause]
  Subsystem3/3(EWPBUflag) -> VTHC_EWPBUflag1_flg/1
  Subsystem1/2(EWPpause) -> [EWP2pause]
  Subsystem2/2(EWPpause) -> [EWP3pause]
  Subsystem1/3(EWPBUflag) -> VTHC_EWPBUflag2_flg/1
  Subsystem2/3(EWPBUflag) -> VTHC_EWPBUflag3_flg/1
  Switch10/1 -> EWP1/1
  [EWP1pause] -> Switch10/2
  [EWP1] -> Switch10/3
  Constant3/1 -> Data Type Conversion5/1
  Data Type Conversion5/1 -> Switch10/1
  [EWP2pause] -> Switch11/2
  Constant4/1 -> Data Type Conversion6/1
  Data Type Conversion6/1 -> Switch11/1
  [EWP2] -> Switch11/3
  Switch11/1 -> EWP2/1
  Switch12/1 -> EWP3/1
  [EWP3pause] -> Switch12/2
  Data Type Conversion7/1 -> Switch12/1
  Constant5/1 -> Data Type Conversion7/1
  [EWP3] -> Switch12/3
  [FWVForceON] -> VTHC_THSysErrlampReq_flg/1  "VTHC_THSysErrlampReq_flg"

== system thc/THC/ThermalControl/THCM_Conctrl/Subsystem4 ==
  sigSetTempZon1St : Inport
  Tamb : Inport  Port=2
  Add1 : Sum
  Add2 : Sum  Inputs=+-
  Constant : Constant  Value=0.5
  Constant1 : Constant  Value=0.5
  Constant2 : Constant
  Constant3 : Constant  Value=0
  Data Type Conversion : DataTypeConversion  OutDataTypeStr=single
  Data Type Conversion1 : DataTypeConversion  OutDataTypeStr=single
  Data Type Conversion2 : DataTypeConversion  OutDataTypeStr=boolean
  Data Type Conversion3 : DataTypeConversion  OutDataTypeStr=boolean
  Relational Operator : RelationalOperator  Operator=<=  OutDataTypeStr=boolean  RndMeth=Simplest
  Relational Operator1 : RelationalOperator  Operator=>  OutDataTypeStr=boolean  RndMeth=Simplest
  Switch : Switch  Criteria=u2 > Threshold
  Switch1 : Switch  Criteria=u2 > Threshold
  Unit Delay : UnitDelay  SampleTime=-1  HasFrameUpgradeWarning=on
  HeatReq : Outport
  wires:
  [sigSetTempZon1St] -> Add1/1
  Constant/1 -> Data Type Conversion/1
  Data Type Conversion/1 -> Add1/2
  Data Type Conversion1/1 -> Add2/2
  Constant1/1 -> Data Type Conversion1/1
  [sigSetTempZon1St] -> Add2/1
  Tamb/1 -> [Tamb]
  [Tamb] -> Relational Operator/1
  Add2/1 -> Relational Operator/2
  Relational Operator/1 -> Switch/2
  Constant2/1 -> Data Type Conversion2/1
  Data Type Conversion2/1 -> Switch/1
  [Tamb] -> Relational Operator1/1
  Add1/1 -> Relational Operator1/2
  Relational Operator1/1 -> Switch1/2
  Constant3/1 -> Data Type Conversion3/1
  Data Type Conversion3/1 -> Switch1/1
  Switch1/1 -> Switch/3
  Unit Delay/1 -> Switch1/3
  Switch/1 -> HeatReq/1, Unit Delay/1
  sigSetTempZon1St/1 -> [sigSetTempZon1St]

== system thc/THC/ThermalControl/THCM_Conctrl/WPTC ==
  WPTC : Inport
  EWP3_Err : Inport  Port=2
  PresetValue : Inport  Port=3
  Constant : Constant  Value=KTHC_ErrHandleEN_flg
  Logical Operator : Logic  AllPortsSameDT=off  OutDataTypeStr=boolean
  Switch : Switch  Criteria=u2 > Threshold
  DataOut : Outport
  wires:
  Logical Operator/1 -> Switch/2
  EWP3_Err/1 -> Logical Operator/1
  Constant/1 -> Logical Operator/2
  PresetValue/1 -> Switch/1
  WPTC/1 -> Switch/3
  Switch/1 -> DataOut/1

== system thc/THC/ThermalControl/THCM_Conctrl/APTC/APTCPIControl ==
  x : Inport
  Reset : Inport  Port=2
  CtrlReset : Inport  Port=3
  VTHC_KpAPTC_K : Inport  Port=4
  VTHC_KiAPTC_K : Inport  Port=5
  Add : Sum
  Add1 : Sum
  Constant : Constant  Value=0
  Equal : RelationalOperator  Operator=~=  OutDataTypeStr=boolean  RndMeth=Simplest
  Logical Operator : Logic  Operator=OR  AllPortsSameDT=off  OutDataTypeStr=boolean
  Product : Product
  Product1 : Product
  Saturation : Saturate  UpperLimit=1  LowerLimit=0
  Switch : Switch  Criteria=u2 > Threshold
  Ts : Gain  Gain=0.1
  Unit Delay : UnitDelay  SampleTime=-1  HasFrameUpgradeWarning=on
  Unit Delay1 : UnitDelay  SampleTime=-1  HasFrameUpgradeWarning=on
  VTHC_APTCP_K : Outport
  VTHC_APTCI_K : Outport  Port=2
  VTHC_APTCU_K : Outport  Port=3
  wires:
  Logical Operator/1 -> Switch/2
  CtrlReset/1 -> Logical Operator/2
  Ts/1 -> Add1/1  "VTHC_APTCI_K"
  Product1/1 -> Ts/1
  Add1/1 -> Unit Delay1/1
  x/1 -> Product1/2, Product/2
  Saturation/1 -> Switch/3
  VTHC_KiAPTC_K/1 -> Product1/1
  VTHC_KpAPTC_K/1 -> Product/1
  Reset/1 -> Equal/1, Unit Delay/1
  Unit Delay1/1 -> Saturation/1
  Switch/1 -> Add1/2, Add/2, VTHC_APTCI_K/1  "VTHC_APTCI_K"
  Add/1 -> VTHC_APTCU_K/1
  Product/1 -> Add/1, VTHC_APTCP_K/1  "VTHC_APTCP_K"
  Constant/1 -> Switch/1
  Equal/1 -> Logical Operator/1
  Unit Delay/1 -> Equal/2

== system thc/THC/ThermalControl/THCM_Conctrl/APTC/APTCPWMControl ==
  Win : Inport
  Chart : Stateflow chart  TreatAsAtomicUnit=on
  Constant : Constant  Value=KTHC_APTCPeriod_cnt
  Constant1 : Constant  Value=KTHC_APTCQminC_W
  Constant43 : Constant  Value=KTHC_APTCPWMEN_flg
  Data Type Conversion : DataTypeConversion  OutDataTypeStr=uint16
  Data Type Conversion1 : DataTypeConversion  OutDataTypeStr=uint16
  Data Type Conversion2 : DataTypeConversion  OutDataTypeStr=uint16
  Out1 : Outport
  wires:
  Data Type Conversion/1 -> Chart/1(Win)
  Constant1/1 -> Data Type Conversion2/1
  Constant/1 -> Data Type Conversion1/1
  Data Type Conversion2/1 -> Chart/3(Wmin)
  Data Type Conversion1/1 -> Chart/2(Tp)
  Chart/1(Wout) -> Out1/1  "Wout"
  Win/1 -> Data Type Conversion/1  "Win"
  Constant43/1 -> Chart/4(KTHC_APTCPWMEN_flg)

== system thc/THC/ThermalControl/THCM_Conctrl/APTC/APTCPWMControl1 ==
  Win : Inport
  Chart : Stateflow chart  TreatAsAtomicUnit=on
  Constant : Constant  Value=KTHC_APTCPeriod_cnt
  Constant1 : Constant  Value=KTHC_APTCQminC_W
  Constant43 : Constant  Value=KTHC_APTCPWMEN_flg
  Data Type Conversion : DataTypeConversion  OutDataTypeStr=uint16
  Data Type Conversion1 : DataTypeConversion  OutDataTypeStr=uint16
  Data Type Conversion2 : DataTypeConversion  OutDataTypeStr=uint16
  Out1 : Outport
  wires:
  Constant43/1 -> Chart/4(KTHC_APTCPWMEN_flg)
  Win/1 -> Data Type Conversion/1  "Win"
  Chart/1(Wout) -> Out1/1  "Wout"
  Data Type Conversion1/1 -> Chart/2(Tp)
  Data Type Conversion2/1 -> Chart/3(Wmin)
  Constant/1 -> Data Type Conversion1/1
  Constant1/1 -> Data Type Conversion2/1
  Data Type Conversion/1 -> Chart/1(Win)

== system thc/THC/ThermalControl/THCM_Conctrl/APTC/APTCPWMControl2 ==
  Win : Inport
  Chart : Stateflow chart  TreatAsAtomicUnit=on
  Constant : Constant  Value=KTHC_APTCPeriod_cnt
  Constant1 : Constant  Value=KTHC_APTCQminC_W
  Constant43 : Constant  Value=KTHC_APTCPWMEN_flg
  Data Type Conversion : DataTypeConversion  OutDataTypeStr=uint16
  Data Type Conversion1 : DataTypeConversion  OutDataTypeStr=uint16
  Data Type Conversion2 : DataTypeConversion  OutDataTypeStr=uint16
  Out1 : Outport
  wires:
  Data Type Conversion/1 -> Chart/1(Win)
  Constant1/1 -> Data Type Conversion2/1
  Constant/1 -> Data Type Conversion1/1
  Data Type Conversion2/1 -> Chart/3(Wmin)
  Data Type Conversion1/1 -> Chart/2(Tp)
  Chart/1(Wout) -> Out1/1  "Wout"
  Win/1 -> Data Type Conversion/1  "Win"
  Constant43/1 -> Chart/4(KTHC_APTCPWMEN_flg)

== system thc/THC/ThermalControl/THCM_Conctrl/APTC/Subsystem ==
  VehSpeed : Inport
  sigSetTempZon1St : Inport  Port=2
  sigSetTempZon2St : Inport  Port=3
  APTCQ : Inport  Port=4
  APTCPID : Inport  Port=5
  1-D Lookup Table : Lookup_n-D  NumberOfTableDimensions=1  BreakpointsForDimension1=ATHC_Qeq_X_kmh  Table=MTHC_Qeq_Y_K  InternalRulePriority=Speed  RndMeth=Simplest  InputSameDT=on
  Abs : Abs
  Add : Sum  Inputs=+-
  Add1 : Sum
  Add2 : Sum
  Add3 : Sum  Inputs=+--
  Add4 : Sum  Inputs=-+
  Compare To Constant : simulink/Logic and Bit Operations/Compare To Constant  relop=>=  const=0  OutDataTypeStr=boolean
  Compare To Constant1 : simulink/Logic and Bit Operations/Compare To Constant  relop=<  const=0  OutDataTypeStr=boolean
  Compare To Constant2 : simulink/Logic and Bit Operations/Compare To Constant  relop=>=  const=0  OutDataTypeStr=boolean
  Compare To Constant4 : simulink/Logic and Bit Operations/Compare To Constant  relop=<  const=0  OutDataTypeStr=boolean
  Constant{,1..5} (6 alike) : Constant  Value=0
  Constant6 : Constant  Value=KTHC_DriverSeatPos_flg
  Constant7 : Constant  Value=KTHC_DriverSeatPos_flg
  Gain : Gain  Gain=-1
  Gain1 : Gain  Gain=2
  Gain2 : Gain  Gain=1/3
  Product : Product
  Relational Operator : RelationalOperator  Operator=>  OutDataTypeStr=boolean  RndMeth=Simplest
  Saturation : Saturate  UpperLimit=KTHC_APTCRiLeMaxDff_W  LowerLimit=KTHC_APTCRiLeMinDff_W
  Saturation1 : Saturate  UpperLimit=KTHC_APTCOneZoneMax_W  LowerLimit=0
  Saturation2 : Saturate  UpperLimit=KTHC_APTCOneZoneMax_W  LowerLimit=0
  Switch{,1..11} (12 alike) : Switch  Criteria=u2 > Threshold
  FD_FrLeAPTC_Cmd : Outport
  FD_FrRiAPTC_Cmd : Outport  Port=2
  FD_RrAPTC_Cmd : Outport  Port=3
  wires:
  [APTCPID] -> Switch7/2
  APTCQ/1 -> [APTCQTemp]
  Switch9/1 -> FD_RrAPTC_Cmd/1
  Constant5/1 -> Switch9/3
  [APTCPID] -> Switch9/2
  Switch5/1 -> Switch9/1
  Switch8/1 -> FD_FrRiAPTC_Cmd/1
  [APTCPID] -> Switch8/2
  Constant4/1 -> Switch8/3
  Constant3/1 -> Switch7/3
  APTCPID/1 -> [APTCPID]
  Switch7/1 -> FD_FrLeAPTC_Cmd/1
  Saturation1/1 -> [VTHC_APTC1stQ_W]
  Constant1/1 -> Switch3/3
  Add2/1 -> Switch4/3
  Add1/1 -> Gain2/1
  [APTCQTemp] -> Relational Operator/2, Add1/1
  Product/1 -> Saturation/1
  [VTHC_APTC1stQ_W] -> Add2/2
  Gain/1 -> Switch3/1
  [VTHC_APTCZone1full_flg] -> Switch5/2
  sigSetTempZon1St/1 -> Add/1
  Compare To Constant1/1 -> Switch3/2
  [Q12] -> Compare To Constant4/1, Add4/1
  [VTHC_APTC1stQ_W] -> Switch6/1
  Switch1/1 -> Switch/1
  Compare To Constant2/1 -> Switch4/2
  Switch3/1 -> Switch2/1
  Abs/1 -> Relational Operator/1, Gain1/1
  Add/1 -> [DTZone]
  [DTZone] -> Product/2
  [Q12] -> Compare To Constant1/1, Gain/1
  [VTHC_APTCZone1full_flg] -> Switch2/2
  Add3/1 -> Saturation2/1
  Relational Operator/1 -> [VTHC_APTCZone1full_flg]
  [Q12] -> Compare To Constant/1, Switch1/1
  sigSetTempZon2St/1 -> Add/2
  [VTHC_APTCZone1full_flg] -> Switch/2
  [APTCFrLeQ] -> Add3/2
  Compare To Constant/1 -> Switch1/2
  Compare To Constant4/1 -> Switch6/2
  Constant2/1 -> Switch5/1
  Add4/1 -> Switch6/3
  [VTHC_APTC1stQ_W] -> Add4/2
  Switch/1 -> [APTCZ1Q]
  Gain2/1 -> Saturation1/1
  Saturation/1 -> Abs/1, [Q12]
  Switch4/1 -> Switch/3
  Switch6/1 -> Switch2/3
  [Q12] -> Compare To Constant2/1, Add2/1
  [APTCFrRiQ] -> Add3/3
  Saturation2/1 -> Switch5/3
  Gain1/1 -> Add1/2
  1-D Lookup Table/1 -> [qeq]
  Constant/1 -> Switch1/3
  [qeq] -> Product/1
  [APTCQTemp] -> Add3/1
  VehSpeed/1 -> 1-D Lookup Table/1
  [VTHC_APTC1stQ_W] -> Switch4/1
  Switch2/1 -> [APTCZ2Q]
  [APTCZ1Q] -> Switch10/1
  [APTCZ2Q] -> Switch10/3
  Constant6/1 -> Switch10/2
  Constant7/1 -> Switch11/2
  [APTCZ1Q] -> Switch11/3
  [APTCZ2Q] -> Switch11/1
  Switch11/1 -> [APTCFrLeQ]
  Switch10/1 -> [APTCFrRiQ]
  [APTCFrLeQ] -> Switch7/1
  [APTCFrRiQ] -> Switch8/1
